simulink model "test_MyPilger5_7V"  (R2025b)
settings: Solver=FixedStepAuto  StartTime=0.0  StopTime=6.36745994232553  FixedStep=0.001611199378  RelTol=1e-3
model workspace (MAT data in the model file):
  c1 = 2.36599978206
  c2 = 1007643.75141
  c3 = 1000070.52701
  c4 = 999985.300894
  fri = 159.462775919
  ges = [0.002 0.004 0.006 0.008 0.01 0.012 0.014 0.016 0.018 0.02 0.022 0.024 ... (66942 elements, 22314x3)]
  j1 = 0.00500803111664
  j2x = 0.00446082292837
  k1 = 1608676.75432
  k2 = 902196412.061
  k3 = 999959312.318
  k4 = 1000025839.46
  m1 = 6903.78290806
  m2 = 499.294055734
  m3 = 249.818133614
  nse = 0.89970043598
  pt = 0.001029670004
  sne = 0.900037480073
values from neighbouring files (symbols this model uses):
  c = [1.685082264734805,1.6814466953741207e-06,0.009999993257493107,0.9000145671384575,0.10000133609148719,0.0020000187958843815,8.47842304562683e-05]    [test.m]
libraries: fl_lib x7, nesl_utility x3, sdl_lib x2, SignalEditorBlockLib x1
settings Model: Creator=alexp  LastModifiedBy=cschmied
settings SolverCC: AlgebraicLoopSolver=TrustRegion
settings DataIOCC: ReturnWorkspaceOutputs=off
settings OptimizationCC: DefaultParameterBehavior=Inlined  OptimizeBlockIOStorage=off  BufferReuse=off  GlobalBufferReuse=off  ExpressionFolding=off  PassReuseOutputArgsThreshold=0.0  LocalBlockOutputs=off  OptimizeDataStoreBuffers=off  BusAssignmentInplaceUpdate=off
settings DebuggingCC: ParameterTunabilityLossMsg=error  UnconnectedInputMsg=warning  UnconnectedOutputMsg=warning  UnconnectedLineMsg=warning  SFUnexpectedBacktrackingDiag=warning  SFNoUnconditionalDefaultTransitionDiag=warning
settings ModelReferenceCC: EnableRefExpFcnMdlSchedulingChecks=on
settings SFSimCC: MATLABDynamicMemAlloc=off
settings RTWCC: GenCodeOnly=on  GenerateReport=on  BuildConfiguration=Debug  LaunchReport=on  GPUComputeCapability=3.5
settings CodeAppCC: ForceParamTrailComments=on  OperatorAnnotations=on  MATLABSourceComments=on  EnableCustomComments=on
settings GRTTargetCC: MultiInstanceErrorCode=Warning  CombineSignalStateStructs=on  SupportVariableSizeSignals=on
settings SimscapeCC: SimscapeLogType=all  SimscapeLogLimitData=off

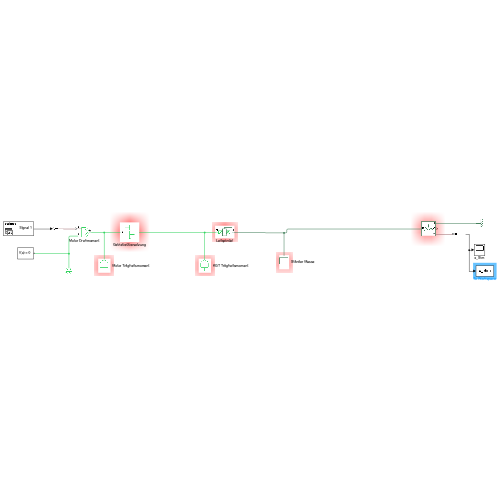
[thumbnail: Simulink's stored preview of the top-level diagram]
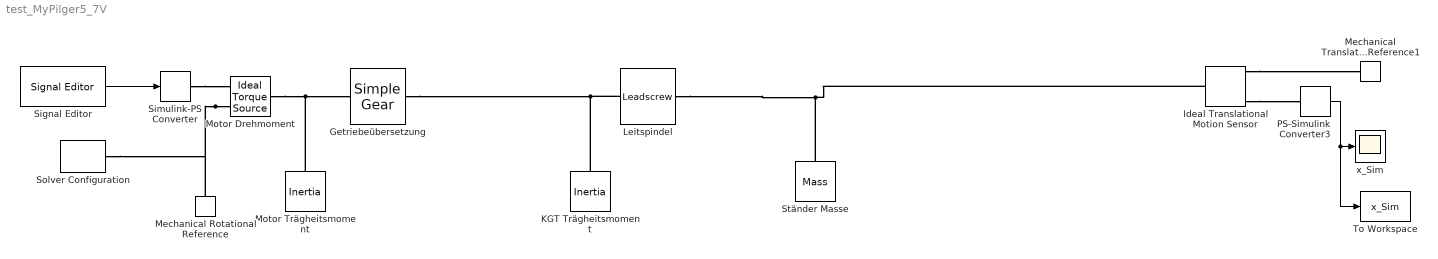
== system test_MyPilger5_7V ==
  Getriebeübersetzung : sdl_lib/Gears/Simple Gear  ratio=c(5)  rotation_direction=3-2*(2)  friction_model=sdl.enum.gear_efficiencies_load.constant  T_noload=0.1 N*m  T_nom=5 N*m  efficiency_nom=0.8  efficiency=c(4)  temperature_TLU=[280, 300, 320] K  load_TLU=[1, 5, 10] N*m  efficiency_TLU=[.95, .9, .85]  efficiency_TLU2=[.85, .8, .75; .95, .9, .85; .85, .8, .7]  w_thr=0.01 rad/s  pwr_thr=0.001 W  enable_backlash=false  hardstop_model=simscape.enum.hardstop.smooth  backlash_distance=1e-3 mm  r_base=0.1 m  transition=1e-4 mm  backlash_stiffness=1e7 N/m  backlash_damping=1e6 N*s/m  coeff_rest=0  v_tol=0.001 m/s  f_tol=0 N  mu_visc=[0,0] N*m/(rad/s)  thermal_mass=50 J/K  temperature_specify=off  temperature_priority=High  temperature=300 K  temperature_nominal_specify=off  temperature_nominal_value=1  temperature_nominal_unit=K  x_backlash_specify=off  x_backlash_priority=None  x_backlash=0 mm  x_backlash_nominal_specify=off  x_backlash_nominal_value=1  x_backlash_nominal_unit=mm  f_hardstop_specify=off  f_hardstop_priority=None  f_hardstop=0 N  f_hardstop_nominal_specify=off  f_hardstop_nominal_value=1  f_hardstop_nominal_unit=N  v_backlash_specify=off  v_backlash_priority=None  v_backlash=0 m/s  v_backlash_nominal_specify=off  v_backlash_nominal_value=1  v_backlash_nominal_unit=m/s
  Ideal Translational Motion Sensor : fl_lib/Mechanical/Mechanical Sensors/Ideal Translational Motion Sensor  reference=foundation.enum.MeasurementReference.difference  acceleration_port=false  velocity_port=true  position_port=true  offset=start_position mm
  KGT Trägheitsmoment : fl_lib/Mechanical/Rotational Elements/Inertia  inertia=c(2) kg*m^2  num_ports=foundation.enum.numPorts2.one  w_specify=off  w_priority=High  w=0 rad/s  w_nominal_specify=off  w_nominal_value=1  w_nominal_unit=rad/s  t_specify=off  t_priority=None  t=0 N*m  t_nominal_specify=off  t_nominal_value=1  t_nominal_unit=N*m
  Leitspindel : sdl_lib/Gears/Rotational- Translational/Leadscrew  Lead=c(6) m  helix_type=1  friction_model=1  friction_parameterization=1  lambda=15 deg  alpha=14.5 deg  fr_coeff=0.002  eff_sn=0.99  eff_ns=0.99  temperature_TLU=[280, 300, 320] K  efficiency_sn_TLU=[.75, .65, .6]  efficiency_ns_TLU=[.5, .45, .4]  pwr_thr=pt W  mu_visc=c(3) N*m/(rad/s)  thermal_mass=50 J/K  temperature_specify=off  temperature_priority=High  temperature=300 K  temperature_nominal_specify=off  temperature_nominal_value=1  temperature_nominal_unit=K
      settings: InternalSimscapePortConfiguration="{\"Bottom\":[],\"Left\":[{\"id\":\"S\",\"label\":\"S\",\"type\":\"foundation.mechanical.rotational.rotational\"}],\"Right\":[{\"id\":\"N\",\"label\":\"N\",\"type\":\"foundation.mechanical.translational.translational\"}],\"Top\":[]}"
  Mechanical Rotational Reference : fl_lib/Mechanical/Rotational Elements/Mechanical Rotational Reference
  Mechanical Translational Reference1 : fl_lib/Mechanical/Translational Elements/Mechanical Translational Reference
  Motor Drehmoment : fl_lib/Mechanical/Mechanical Sources/Ideal Torque Source
  Motor Trägheitsmoment : fl_lib/Mechanical/Rotational Elements/Inertia  inertia=c(7) kg*m^2  num_ports=foundation.enum.numPorts2.one  w_specify=off  w_priority=High  w=0 rad/s  w_nominal_specify=off  w_nominal_value=1  w_nominal_unit=rad/s  t_specify=off  t_priority=None  t=0 N*m  t_nominal_specify=off  t_nominal_value=1  t_nominal_unit=N*m
  PS-Simulink Converter3 : nesl_utility/PS-Simulink Converter  PhysicalDomain=network_engine_domain  SubClassName=ps_output  LeftPortType=input  RightPortType=output  PseudoPeriodic=off  Frequencies=[]  VectorFormat=1-D array  Unit=mm  AffineConversion=off
  Signal Editor : SignalEditorBlockLib/Signal Editor  FileName=testdataset.mat  ActiveScenario=dataset  ActiveSignal=2026-01-31_16-44-26_MyPilger5_1_F6000  IsBus=off  OutputBusObjectStr=Bus: BusObject  SampleTime=0  Interpolate=off  ZeroCross=off  OutputAfterFinalValue=Setting to zero  Unit=inherit  PreserveSignalName=on  ApplySigPropsToAllScenarios=on  ApplySigPropsToAllSignals=off  SignalPropertySource=Dialog parameters
  Simulink-PS Converter : nesl_utility/Simulink-PS Converter  PhysicalDomain=network_engine_domain  SubClassName=ps_input  LeftPortType=input  RightPortType=output  PseudoPeriodic=off  Frequencies=[]  NoiseDistribution=none  NoiseParameters=[]  Unit=N*m  AffineConversion=off  FilteringAndDerivatives=filter  SimscapeFilterOrder=2  InputFilterTimeConstant=0.0001  UdotUserProvided=0
  Solver Configuration : nesl_utility/Solver Configuration  PhysicalDomain=network_engine_domain  SubClassName=solver  LeftPortType=input  RightPortType=generic  Tones=[]  Harmonics=[]  SimulateNoise=off  Profile=off  UseLocalSampling=off  EnableSwitchedLinearOptims=on  FrequencyDomain=off  UseCCode=off  RelTol=0.001  AbsTol=1e-06  MinStep=1e-09  ToWorkspace=off  RevertToSquareIcSolve=off  NumHomotopyIterations=100  PhasorMode=off  PhasorModeNumHarmonics=1  ConsistencySolver=NEWTON_FTOL  IndexReductionMethod=DerivativeReplacement  DoDC=off  ResidualTolerance=1e-09  ConsistencyTolSource=GLOBAL  ConsistencyAbsTol=0.001  ConsistencyRelTol=0.001  ConsistencyTolFactor=0.001  UseLocalSolver=off  LocalSolverChoice=NE_BACKWARD_EULER_ADVANCER  ResolveIndetEquations=on  FunctionEvalNumThread=1  LocalSolverSampleTime=0.001  DoFixedCost=off  MaxNonlinIter=3  MaxModeIter=2  ComputeImpulses=off  ImpulseIterations=2  LinearAlgebra=Sparse  LinearAlgebraNumThread=0  EquationFormulation=NE_TIME_EF  DelaysMemoryBudget=1024  AutomaticFiltering=on  FilteringTimeConstant=0.001  PartitionStorageMethod=AS_NEEDED  PartitionMemoryBudget=1024  PartitionMethod=FAST  MultibodyUseLocalSolver=off  MultibodyLocalSolverChoice=ODE1  MultibodyLocalSolverSampleTime=0.001
  Ständer Masse : fl_lib/Mechanical/Translational Elements/Mass  mass=c(1) kg  num_ports=foundation.enum.numPorts2.one  v_specify=off  v_priority=High  v=0 m/s  v_nominal_specify=off  v_nominal_value=1  v_nominal_unit=m/s  f_specify=off  f_priority=None  f=0 N  f_nominal_specify=off  f_nominal_value=1  f_nominal_unit=N
  To Workspace : ToWorkspace  VariableName=x_Sim  SampleTime=0.001611199378
      settings: Save2DSignal=2-D array (concatenate along first dimension)
  "x_Sim " : Scope
      settings: Title=Positionsverlauf aus simulierter Fahrt  ActiveDisplayYMinimum=-0.28197  ActiveDisplayYMaximum=0.24435  YLabel=Position [mm]
  wires:
  PS-Simulink Converter3/1 -> To Workspace/1, "x_Sim "/1
  Signal Editor/1 -> Simulink-PS Converter/1
  connections:
  Ständer Masse/LConn1 -- Leitspindel/RConn1 -- Ideal Translational Motion Sensor/LConn1
  Motor Trägheitsmoment/LConn1 -- Getriebeübersetzung/LConn1 -- Motor Drehmoment/LConn1
  Leitspindel/LConn1 -- Getriebeübersetzung/RConn1 -- KGT Trägheitsmoment/LConn1
  Motor Drehmoment/RConn2 -- Mechanical Rotational Reference/LConn1 -- Solver Configuration/RConn1
  Ideal Translational Motion Sensor/RConn1 -- Mechanical Translational Reference1/LConn1
  Ideal Translational Motion Sensor/RConn3 -- PS-Simulink Converter3/LConn1
  Simulink-PS Converter/RConn1 -- Motor Drehmoment/RConn1
